simulink model "IFOC_SPVM"  (Simulink 8.3)
settings: Solver=ode23tb  SolverMode=SingleTasking  StartTime=0.0  StopTime=3
InitFcn:
  | assignin('base','Ts',[2e-6]); load power_acdrive_init;
undefined symbols (not defined in the file): Tlim
libraries: powerlib x7
Description:
  | The Model initialization function Callback automatically
  | 
  | sets the sample time  to 2e-6 sec.  and loads the initial
  | 
  | states vector xInitial. The initial state vector is saved in the
  | 
  | power_acdrive_init.mat file.
  | 
  | 
  | 
  | Check  the Initial state checkbox in the Simulation
  | 
  | parameters/Workspace I/O to start in steady state with a
  | 
  | speed of 120 rad/s and a torque of 0 N.m/s,
settings Model: Creator=Hoang Lehuy, Laval University  LastModifiedBy=Keshav  ExtModeTrigMode=oneshot  ExtModeArmWhenConnect=off  ExtModeAutoUpdateStatusClock=off
settings DataIOCC: LimitDataPoints=off  SaveFinalState=on  SaveFormat=StructureWithTime  SaveOutput=off  SaveTime=off  SignalLoggingName=sigsOut
settings OptimizationCC: BlockReduction=off  ExpressionDepthLimit=2147483647  InitFltsAndDblsToZero=on
settings DebuggingCC: SaveWithParameterizedLinksMsg=none  CheckExecutionContextPreStartOutputMsg=on  CheckExecutionContextRuntimeOutputMsg=on  SignalResolutionControl=TryResolveAllWithWarning  SolverPrmCheckMsg=none  MultiTaskDSMMsg=warning  MultiTaskCondExecSysMsg=none  FcnCallInpInsideContextMsg=UseLocalSettings  UnconnectedOutputMsg=none
settings HardwareCC: TargetUnknown=on
settings RTWCC: TemplateMakefile=grt_vc.tmf  IncludeERTFirstTime=on
settings GRTTargetCC: TargetFcnLib=ansi_tfl_tmw.mat

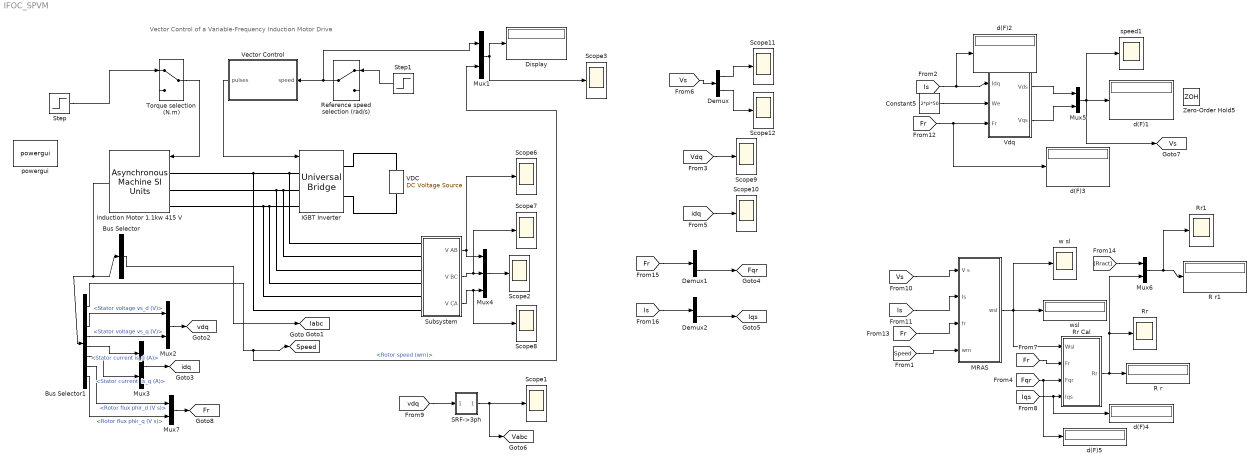
== system IFOC_SPVM ==
  note: Vector Control of a Variable-Frequency Induction Motor Drive
  Bus Selector : BusSelector  OutputSignals=Stator measurements.Stator current is_a (A),Stator measurements.Stator current is_b (A),Stator measurements.Stator current is_c (A)  OutputAsBus=on
  Bus Selector1 : BusSelector  OutputSignals="Mechanical.Rotor speed (wm),Mechanical.Electromagnetic torque Te (N*m),Stator measurements.Stator voltage vs_d (V),Stator measurements.Stator voltage vs_q (V),Stator measurements.Stator current is_d (A),Stator measurements.Stator current  is_q (A),Rotor measurements.Rotor flux phir_d (V s),Rotor measurements.Rotor flux phir_q (V s)"
  Constant5 : Constant  Value=2*pi*50
  Demux : Demux  Outputs=2
  Demux1 : Demux  Outputs=2
  Demux2 : Demux  Outputs=2
  Display : Display
  IGBT Inverter : powerlib/Power Electronics/Universal Bridge  Arms=3  SnubberResistance=1000  SnubberCapacitance=inf  Device=IGBT / Diodes  Ron=1e-3  Lon=0  ForwardVoltages="[  0.8  0.8  ]"  ForwardVoltage=.8  GTOparameters=[ 1e-6 , 1e-6 ]  IGBTparameters=[ 1e-6 , 2e-6 ]  Measurements=None  Measurements_2=None  converterType=Rectifier
  Induction Motor 1.1kw 415 V : powerlib/Machines/Asynchronous Machine SI Units  PresetModel=No  MechanicalLoad=Torque Tm  ShowDetailedParameters=on  RotorType=Squirrel-cage  ReferenceFrame=Synchronous  Units=SI  MeasurementBus=off  NominalParameters=[ 1.1e3,415, 50 ]  Stator=[6.03 0.0299]  Rotor=[12 0.0299]  Cage1=[ 0.022 0.226/377]  Cage2=[ 0.022 0.226/377]  Lm=0.4893  Mechanical="[0.011787  0.0027 2 ]"  PolePairs=2  InitialConditions="[ 1, 0 ,  0 , 0 , 0 , 0 , 0 , 0 ]"  SimulateSaturation=off  Saturation=[9.9249,19.6672,38.0377,51.3988,69.2824,105.1337,152.5532,214.2421,303.1917;230, 322, 414, 460, 506, 552, 598, 644, 690]  LoadFlowParameters=0  TsPowergui=0  TsBlock=-1  IterativeModel=Trapezoidal non iterative  Pmec=0
  MRAS : Subsystem  mask{Kp=100, Ki=50}
      mask prompts: Kp "Proportional Gain (Kp)"; Ki "Integral Gain (Ki)"
  Mux{1..3,5..7} (6 alike) : Mux  Inputs=2
  Mux4 : Mux  Inputs=3
  R r : Display
  R r1 : Display
  Reference speed selection (rad/s) : ManualSwitch
  Rr : Scope
      settings: TimeRange=2  YMin=0  YMax=1.4  SaveName=ScopeData2  MaxDataPoints=20000  Decimation=20
  Rr Cal : Subsystem
  Rr1 : Scope
      settings: TimeRange=2  YMin=12.14  YMax=12.17  SaveName=Resistance  MaxDataPoints=20000  Decimation=20
  SRF->3ph : Subsystem  AncestorBlock=plecslib_extras/Transformations/SRF->3ph  mask(Transformation SRF->3ph){}
      mask help:
      | Transforms a two-dimensional vector in the stationary reference frame into a three-phase signal:
      | [alpha beta] -> [a b c]
      mask Help: web(['file:///' fullfile(plecsdoc, 'alphabeta2abc.html')])
      mask Display: plot([0 100],[0 100], [0.5 3 4 4 5 4 3 1 0 0 1 4]*4+36,[7 7 6 3 2 3 2 2 3 4 5 5]*4, [0 1 3 4 4 3 1 0 0 0]*4+60,[6 7 7 6 3 2 2 3 2 10]*4, [4 3 1 0 0 1 3 4]*4+84,[6 7 7 6 3 2 2 3]*4, [5 3 1 0 0 1 3 5]*4,[7 2 2 3 6 7 7 2]*4+62, [0 0 1 3 4 4 3 2 3 4 4 3 1]*4+35,[0 8 9 9 8 7 6 6 6 5 3 2 2]*4+62 )
  Scope{1..3,6..12} (10 alike) : Scope
      Scope1 settings: TimeRange=0.5  YMin=-800  YMax=700  Decimation=20  SampleTime=5e-6
      Scope10 settings: TimeRange=0.5  YMin=1.5  YMax=4.5  SaveName=ScopeData9  Decimation=20  SampleTime=5e-6
      Scope11 settings: TimeRange=0.5  YMin=230  YMax=360  SaveName=ScopeData10  Decimation=20  SampleTime=5e-6
      Scope12 settings: TimeRange=0.5  YMin=-900  YMax=800  SaveName=ScopeData11  Decimation=20  SampleTime=5e-6
      Scope2 settings: TimeRange=0.5  YMin=-100  YMax=700  SaveName=ScopeData15  Decimation=20  SampleTime=5e-6
      Scope3 settings: TimeRange=0.5  YMin=-100  YMax=700  SaveName=ScopeData7  Decimation=20  SampleTime=5e-6
      Scope6 settings: TimeRange=0.5  YMin=-50  YMax=700  SaveName=ScopeData4  Decimation=20  SampleTime=5e-6
      Scope7 settings: TimeRange=0.5  YMin=-100  YMax=700  SaveName=ScopeData5  Decimation=20  SampleTime=5e-6
      Scope8 settings: TimeRange=0.5  YMin=-100  YMax=700  SaveName=ScopeData6  Decimation=20  SampleTime=5e-6
      Scope9 settings: TimeRange=0.5  YMin=-500  YMax=500  SaveName=ScopeData8  Decimation=20  SampleTime=5e-6
  Step : Step  Time=0  Before=7.5  After=7.5  SampleTime=0
  Step1 : Step  Time=0  Before=148.2  After=148.2  SampleTime=0
  Subsystem : Subsystem
  Torque selection (N.m) : ManualSwitch
  VDC : powerlib/Electrical Sources/DC Voltage Source  Description=source block  Amplitude=700  Measurements=None
      settings: AttributesFormatString=\n
  Vdq : Subsystem
  Vector Control : Subsystem
  Zero-Order Hold5 : ZeroOrderHold  SampleTime=0.1e-3
  d(F){1..5} (5 alike) : Display
  powergui : powerlib/powergui  Priority=1  SimulationMode=Continuous  SolverType=Tustin  SampleTime=50e-6  frequency=60  SPID=off  DisableSnubberDevices=off  DisableRonSwitches=off  DisableVfSwitches=off  SwTol=0  Interpol=off  DisplayEquations=off  Ts=0  methode=off  frequencyindice=50  Pbase=100e6  ErrMax=1e-4  Iterations=50  UnitsV=kV  UnitsW=MW  FunctionMessages=off  echomessages=off  HookPort=off  EnableUseOfTLC=off  x0status=blocks  RestoreLinks=warning  ResistiveCurrentMeasurement=off  Frange=[0:2:500]  Ylog=off  Xlog=on  ShowGrid=off  save=off  variable=ZData  structure=0  ZoomFFT=off  StartTime=0.0  cycles=1  DisplayStyle=1  fundamental=60  FreqAxis=off  MaxFrequency=1000  frequencyindicesteady=1  RmsSteady=1  display=off
  speed1 : Scope
      settings: TimeRange=2  YMin=-250  YMax=350  MaxDataPoints=20000  Decimation=20
  w sl : Scope
      settings: TimeRange=2  YMin=0  YMax=1.4  SaveName=ScopeData12  MaxDataPoints=20000  Decimation=20
  wsl : Display
  tag scope: Fqr=global, Fr=global, Iabc=global, Iqs=global, Speed=global, Vabc=global, Vs=global, idq=global, vdq=global
  wires:
  Torque selection (N.m)/1 -> Induction Motor 1.1kw 415 V/1
  Reference speed selection (rad/s)/1 -> Vector Control/1(speed), Mux1/1
  Induction Motor 1.1kw 415 V/1 -> Bus Selector1/1, Bus Selector/1
  Bus Selector/1 -> [Iabc]
  Bus Selector1/1 -> [Speed], Mux1/2  "<Rotor speed (wm)>"
  Mux1/1 -> Display/1, Scope3/1
  Vector Control/1(pulses) -> IGBT Inverter/1
  Mux2/1 -> [vdq]
  Mux3/1 -> [idq]
  Step1/1 -> Reference speed selection (rad/s)/1
  Step/1 -> Torque selection (N.m)/1
  Subsystem/1(V AB) -> Mux4/1, Scope6/1
  Subsystem/2(V BC) -> Mux4/2, Scope7/1
  Subsystem/3(V CA) -> Mux4/3, Scope8/1
  [Vdq] -> Scope9/1
  [idq] -> Scope10/1
  [Vs] -> Demux/1
  Demux/1 -> Scope11/1
  Demux/2 -> Scope12/1
  Mux4/1 -> Scope2/1
  Bus Selector1/3 -> Mux2/1  "<Stator voltage vs_d (V)>"
  Bus Selector1/4 -> Mux2/2  "<Stator voltage vs_q (V)>"
  Bus Selector1/5 -> Mux3/1  "<Stator current is_d (A)>"
  Bus Selector1/6 -> Mux3/2  "<Stator current  is_q (A)>"
  [Is] -> d(F)2/1, Vdq/1(Idq)
  Constant5/1 -> Vdq/2(We)
  Mux5/1 -> d(F)1/1, speed1/1, [Vs]
  Vdq/1(Vds) -> Mux5/1
  Vdq/2(Vqs) -> Mux5/2
  [Fr] -> d(F)3/1, Vdq/3(Fr)
  Bus Selector1/7 -> Mux7/1  "<Rotor flux phir_d (V s)>"
  Bus Selector1/8 -> Mux7/2  "<Rotor flux phir_q (V s)>"
  Mux7/1 -> [Fr]
  SRF->3ph/1(abc) -> Scope1/1, [Vabc]
  [vdq] -> SRF->3ph/1(alpha beta)
  [Vs] -> MRAS/1(V s)
  [Is] -> MRAS/2(Is)
  [Fr] -> MRAS/3(fr)
  MRAS/1(wsl) -> wsl/1, w sl/1, Rr Cal/1(Wsl)
  [Speed] -> MRAS/4(wm)
  [Fr] -> Rr Cal/2(Fr)
  [Fqr] -> Rr Cal/3(Fqr), d(F)5/1
  [Iqs] -> Rr Cal/4(Iqs), d(F)4/1
  Rr Cal/1(Rr) -> R r/1, Rr/1, Mux6/2
  [Rract] -> Mux6/1
  Mux6/1 -> R r1/1, Rr1/1
  [Fr] -> Demux1/1
  Demux1/2 -> [Fqr]
  [Is] -> Demux2/1
  Demux2/2 -> [Iqs]
  connections:
  IGBT Inverter/RConn2 -- VDC/LConn1
  Induction Motor 1.1kw 415 V/LConn3 -- IGBT Inverter/LConn3 -- Subsystem/LConn4 -- Subsystem/LConn5
  IGBT Inverter/LConn1 -- Subsystem/LConn1 -- Induction Motor 1.1kw 415 V/LConn1 -- Subsystem/LConn6
  IGBT Inverter/RConn1 -- VDC/RConn1
  Induction Motor 1.1kw 415 V/LConn2 -- IGBT Inverter/LConn2 -- Subsystem/LConn2 -- Subsystem/LConn3

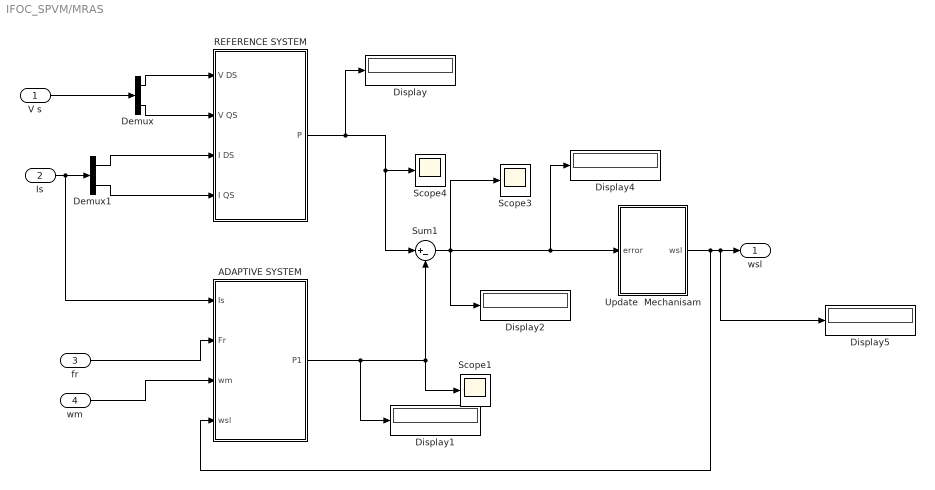
== system IFOC_SPVM/MRAS ==
  V s : Inport
  Is : Inport  Port=2
  fr : Inport  Port=3
  wm : Inport  Port=4
  ADAPTIVE SYSTEM : Subsystem
  Demux : Demux  Outputs=2
  Demux1 : Demux  Outputs=2
  Display{,1..2,4..5} (5 alike) : Display
  REFERENCE SYSTEM : Subsystem
  Scope1 : Scope
      settings: YMin=-1  YMax=1
  Scope3 : Scope
      settings: YMin=-1  YMax=1  SaveName=ScopeData16
  Scope4 : Scope
      settings: YMin=-1  YMax=1  SaveName=ScopeData4
  Sum1 : Sum  Inputs=|+-  SaturateOnIntegerOverflow=on  InputSameDT=on  OutDataTypeStr=Inherit: Same as first input
  Update  Mechanisam : Subsystem
  wsl : Outport
  wires:
  Demux/1 -> REFERENCE SYSTEM/1(V DS)
  Demux/2 -> REFERENCE SYSTEM/2(V QS)
  Demux1/1 -> REFERENCE SYSTEM/3(I DS)
  Demux1/2 -> REFERENCE SYSTEM/4(I QS)
  REFERENCE SYSTEM/1(P) -> Display/1, Sum1/1, Scope4/1
  ADAPTIVE SYSTEM/1(P1) -> Sum1/2, Scope1/1, Display1/1
  Is/1 -> Demux1/1, ADAPTIVE SYSTEM/1(Is)
  V s/1 -> Demux/1
  Sum1/1 -> Display2/1, Scope3/1, Update  Mechanisam/1(error), Display4/1
  fr/1 -> ADAPTIVE SYSTEM/2(Fr)
  wm/1 -> ADAPTIVE SYSTEM/3(wm)
  Update  Mechanisam/1(wsl) -> ADAPTIVE SYSTEM/4(wsl), wsl/1, Display5/1

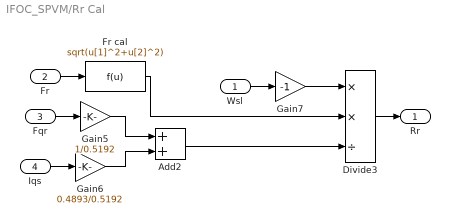
== system IFOC_SPVM/Rr Cal ==
  Wsl : Inport
  Fr : Inport  Port=2
  Fqr : Inport  Port=3
  Iqs : Inport  Port=4
  Add2 : Sum
  Divide3 : Product  Inputs=**/
  Fr cal : Fcn  Expr=sqrt(u[1]^2+u[2]^2)
  Gain5 : Gain  Gain=1/0.5192  SaturateOnIntegerOverflow=on  OutDataTypeStr=Inherit: Same as input  ParamDataTypeStr=Inherit: Same as input
  Gain6 : Gain  Gain=0.4893/0.5192  SaturateOnIntegerOverflow=on  OutDataTypeStr=Inherit: Same as input  ParamDataTypeStr=Inherit: Same as input
  Gain7 : Gain  Gain=-1  SaturateOnIntegerOverflow=on  OutDataTypeStr=Inherit: Same as input  ParamDataTypeStr=Inherit: Same as input
  Rr : Outport
  wires:
  Gain5/1 -> Add2/1
  Gain6/1 -> Add2/2
  Add2/1 -> Divide3/3
  Gain7/1 -> Divide3/1
  Fr cal/1 -> Divide3/2
  Fr/1 -> Fr cal/1
  Wsl/1 -> Gain7/1
  Divide3/1 -> Rr/1
  Fqr/1 -> Gain5/1
  Iqs/1 -> Gain6/1

== system IFOC_SPVM/SRF->3ph ==
  alpha beta : Inport  PortDimensions=2
  Mux : Mux  Inputs=3
  a : Fcn  Expr=u[1]
  b : Fcn  Expr=(-u[1]+sqrt(3)*u[2])/2
  c : Fcn  Expr=(-u[1]-sqrt(3)*u[2])/2
  abc : Outport
  wires:
  a/1 -> Mux/1
  b/1 -> Mux/2
  c/1 -> Mux/3
  Mux/1 -> abc/1
  alpha beta/1 -> b/1, a/1, c/1

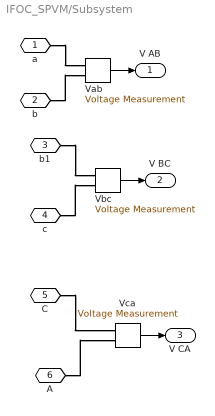
== system IFOC_SPVM/Subsystem ==
  Vab : powerlib/Measurements/Voltage Measurement  Tag=PoWeRsYsTeMmEaSuReMeNt  PhasorSimulation=off  OutputType=Magnitude  PSBequivalent=0
  Vbc : powerlib/Measurements/Voltage Measurement  Tag=PoWeRsYsTeMmEaSuReMeNt  PhasorSimulation=off  OutputType=Magnitude  PSBequivalent=0
  Vca : powerlib/Measurements/Voltage Measurement  Tag=PoWeRsYsTeMmEaSuReMeNt  PhasorSimulation=off  OutputType=Magnitude  PSBequivalent=0
  a : PMIOPort  Port=1  Side=Left
  b : PMIOPort  Port=2  Side=Left
  b1 : PMIOPort  Port=3  Side=Left
  c : PMIOPort  Port=4  Side=Left
  C : PMIOPort  Port=5  Side=Left
  A : PMIOPort  Port=6  Side=Left
  V AB : Outport
  V BC : Outport  Port=2
  V CA : Outport  Port=3
  wires:
  Vab/1 -> V AB/1
  Vbc/1 -> V BC/1
  Vca/1 -> V CA/1
  connections:
  a/RConn1 -- Vab/LConn1
  b/RConn1 -- Vab/LConn2
  b1/RConn1 -- Vbc/LConn1
  c/RConn1 -- Vbc/LConn2
  C/RConn1 -- Vca/LConn1
  A/RConn1 -- Vca/LConn2

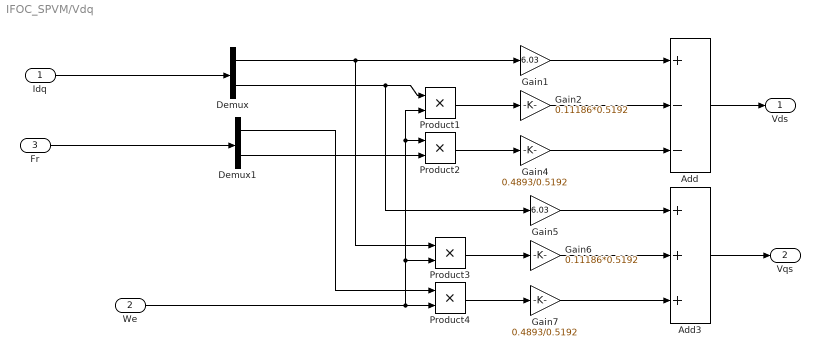
== system IFOC_SPVM/Vdq ==
  Idq : Inport
  We : Inport  Port=2
  Fr : Inport  Port=3
  Add : Sum  Inputs=+--
  Add3 : Sum  Inputs=+++
  Demux : Demux  Outputs=2
  Demux1 : Demux  Outputs=2
  Gain1 : Gain  Gain=6.03
  Gain2 : Gain  Gain=0.11186*0.5192
  Gain4 : Gain  Gain=0.4893/0.5192
  Gain5 : Gain  Gain=6.03
  Gain6 : Gain  Gain=0.11186*0.5192
  Gain7 : Gain  Gain=0.4893/0.5192
  Product{1..4} (4 alike) : Product  RndMeth=Zero
  Vds : Outport
  Vqs : Outport  Port=2
  wires:
  Idq/1 -> Demux/1
  Demux/1 -> Gain1/1, Product3/1
  Demux/2 -> Product1/1, Gain5/1
  Product1/1 -> Gain2/1
  Fr/1 -> Demux1/1
  Demux1/2 -> Product2/2
  Product2/1 -> Gain4/1
  Gain1/1 -> Add/1
  Gain2/1 -> Add/2
  Gain4/1 -> Add/3
  Product3/1 -> Gain6/1
  Product4/1 -> Gain7/1
  Demux1/1 -> Product4/1
  Gain5/1 -> Add3/1
  Gain6/1 -> Add3/2
  Gain7/1 -> Add3/3
  Add/1 -> Vds/1
  Add3/1 -> Vqs/1
  We/1 -> Product1/2, Product2/1, Product3/2, Product4/2

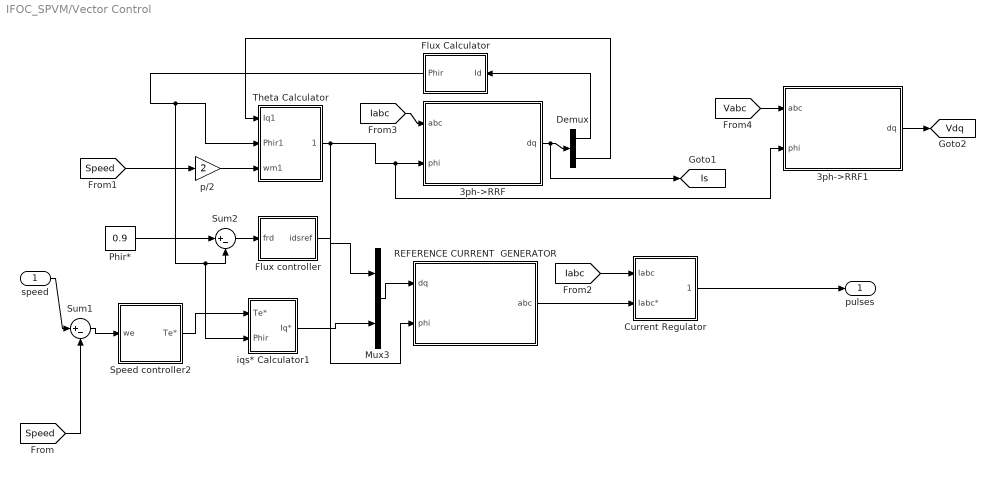
== system IFOC_SPVM/Vector Control ==
  speed : Inport
  " Flux controller" : Subsystem  Description=flux controller  mask(PI controller){Kp=10, Ki=100, MaskParam3=0}
      mask prompts: Kp "proportional gain"; Ki "Integral gain"; MaskParam3 "current limit"
      mask help: flux controller
      settings: ErrorFcn=flux controller
  3ph->RRF : Subsystem  mask(Transformation 3ph->RRF){}
      mask help:
      | Transforms a three-phase signal into a two-dimensional vector in a rotating reference frame. The rotation angle in radians of the rotating reference frame is determined by the second input:
      | [a b c], phi -> [d q]
      mask Help: web(['file:///' fullfile(plecsdoc, 'abc2dq.html')])
      mask Display:
      | plot(-30, -65, 150, 150)
      | plot([0 0 0 100],[0 100 50 50])
      | plot([0:5:100],[50+50.*sin([0:5:100]*2*pi/100)])
      | plot([0:5:100],[50+50.*sin(([0:5:100]*2*pi/100)+(2*pi/3))])
      | port_label('input',1,'ABC')
      | port_label('input',2,'Theta')
      | port_label('output',1,'DQ*')
  3ph->RRF1 : Subsystem  mask(Transformation 3ph->RRF){}
      mask help:
      | Transforms a three-phase signal into a two-dimensional vector in a rotating reference frame. The rotation angle in radians of the rotating reference frame is determined by the second input:
      | [a b c], phi -> [d q]
      mask Help: web(['file:///' fullfile(plecsdoc, 'abc2dq.html')])
      mask Display:
      | plot(-30, -65, 150, 150)
      | plot([0 0 0 100],[0 100 50 50])
      | plot([0:5:100],[50+50.*sin([0:5:100]*2*pi/100)])
      | plot([0:5:100],[50+50.*sin(([0:5:100]*2*pi/100)+(2*pi/3))])
      | port_label('input',1,'ABC')
      | port_label('input',2,'Theta')
      | port_label('output',1,'DQ*')
  Current Regulator : Subsystem  mask(Regulateur de courant a hysteresis){h=0.2}
      mask prompts: h "Hysteresis band (A)"
  Demux : Demux  Outputs=2
  Flux Calculator : Subsystem  mask(Flux Calcultation){}
      mask init:
      | NF=0.44572610323020e-6;
      | DF=[1 -0.99998715486734];
  Mux3 : Mux  Inputs=2
  Phir* : Constant  Value=0.9
  REFERENCE CURRENT  GENERATOR : Subsystem  mask(Transformation RRF->3ph){}
      mask help:
      | Transforms a two-dimensional vector in a rotating reference frame into a three-phase signal. The rotation angle in radians of the rotating reference frame is determined by the second input:
      | [d q], phi -> [a b c]
      mask Help: web(['file:///' fullfile(plecsdoc, 'dq2abc.html')])
      mask Display:
      | plot(-30, -65, 150, 150)
      | plot([0 0 0 100],[0 100 50 50])
      | plot([0:5:100],[50+50.*sin([0:5:100]*2*pi/100)])
      | plot([0:5:100],[50+50.*sin(([0:5:100]*2*pi/100)+(2*pi/3))])
      | plot([0:5:100],[50+50.*sin(([0:5:100]*2*pi/100)-(2*pi/3))])
      | port_label('input',1,'IDQ*')
      | port_label('input',2,'Theta')
      | port_label('output',1,'Iabc*')
  Speed controller2 : Subsystem  mask(PI controller){Kp=0.35, Ki=2.5, Tlim=0}
      mask prompts: Kp "Proportional gain (Kp)"; Ki "Integral gain (Ki)"; Tlim "Torque Limit"
      mask help: Proportional-Integral Speed Controller
      mask Display: plot(0,0,100,100,[35,35,65],[70,30,30],[35,65],[45,60])
  Sum1 : Sum  Inputs=|+-  SaturateOnIntegerOverflow=on  InputSameDT=on  OutDataTypeStr=Inherit: Same as first input
  Sum2 : Sum  Inputs=|+-  SaturateOnIntegerOverflow=on  InputSameDT=on  OutDataTypeStr=Inherit: Same as first input
  Theta Calculator : Subsystem
  iqs* Calculator1 : Subsystem
  p/2 : Gain  Gain=2  SaturateOnIntegerOverflow=on  OutDataTypeStr=Inherit: Same as input  ParamDataTypeStr=Inherit: Same as input
  pulses : Outport
  tag scope: Is=global, Vdq=global
  wires:
  Flux Calculator/1(Phir) -> Theta Calculator/2(Phir1), Sum2/2, iqs* Calculator1/2(Phir)
  [Iabc] -> Current Regulator/1(Iabc)
  [Iabc] -> 3ph->RRF/1(abc)
  Current Regulator/1(Pulses) -> pulses/1
  Sum1/1 -> Speed controller2/1(we)
  speed/1 -> Sum1/1
  [Speed] -> Sum1/2
  Speed controller2/1(Te*) -> iqs* Calculator1/1(Te*)
  Theta Calculator/1(theta1) -> 3ph->RRF/2(phi), 3ph->RRF1/2(phi), REFERENCE CURRENT  GENERATOR/2(phi)
  [Speed] -> p/2/1
  p/2/1 -> Theta Calculator/3(wm1)
  3ph->RRF/1(dq) -> Demux/1, [Is]
  Demux/1 -> Flux Calculator/1(Id)
  Demux/2 -> Theta Calculator/1(Iq1)
  " Flux controller"/1(idsref) -> Mux3/1
  iqs* Calculator1/1(Iq*) -> Mux3/2
  Mux3/1 -> REFERENCE CURRENT  GENERATOR/1(dq)
  REFERENCE CURRENT  GENERATOR/1(abc) -> Current Regulator/2(Iabc*)
  Phir*/1 -> Sum2/1
  Sum2/1 -> " Flux controller"/1(frd)
  [Vabc] -> 3ph->RRF1/1(abc)
  3ph->RRF1/1(dq) -> [Vdq]

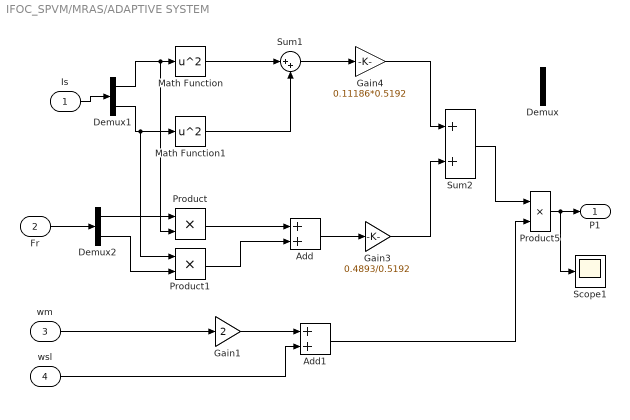
== system IFOC_SPVM/MRAS/ADAPTIVE SYSTEM ==
  Is : Inport
  Fr : Inport  Port=2
  wm : Inport  Port=3
  wsl : Inport  Port=4
  Add : Sum
  Add1 : Sum
  Demux : Demux  Outputs=2
  Demux1 : Demux  Outputs=2
  Demux2 : Demux  Outputs=2
  Gain1 : Gain  Gain=2  SaturateOnIntegerOverflow=on  OutDataTypeStr=Inherit: Same as input  ParamDataTypeStr=Inherit: Same as input
  Gain3 : Gain  Gain=0.4893/0.5192  SaturateOnIntegerOverflow=on  OutDataTypeStr=Inherit: Same as input  ParamDataTypeStr=Inherit: Same as input
  Gain4 : Gain  Gain=0.11186*0.5192  SaturateOnIntegerOverflow=on  OutDataTypeStr=Inherit: Same as input  ParamDataTypeStr=Inherit: Same as input
  Math Function : Math  Operator=square  SaturateOnIntegerOverflow=on
  Math Function1 : Math  Operator=square  SaturateOnIntegerOverflow=on
  Product : Product  RndMeth=Zero
  Product1 : Product  RndMeth=Zero
  Product5 : Product  SaturateOnIntegerOverflow=on  InputSameDT=on  OutDataTypeStr=Inherit: Same as first input
  Scope1 : Scope
      settings: YMin=-1  YMax=1  SaveName=ScopeData3
  Sum1 : Sum  Inputs=|++  SaturateOnIntegerOverflow=on  InputSameDT=on  OutDataTypeStr=Inherit: Same as first input
  Sum2 : Sum  SaturateOnIntegerOverflow=on  InputSameDT=on  OutDataTypeStr=Inherit: Same as first input
  P1 : Outport
  wires:
  Demux1/2 -> Math Function1/1, Product1/1
  Gain4/1 -> Sum2/1
  Sum1/1 -> Gain4/1
  Gain3/1 -> Sum2/2
  Sum2/1 -> Product5/1
  Product5/1 -> P1/1, Scope1/1
  Demux1/1 -> Math Function/1, Product/2
  Math Function/1 -> Sum1/1
  Math Function1/1 -> Sum1/2
  Is/1 -> Demux1/1
  Fr/1 -> Demux2/1
  Demux2/1 -> Product/1
  Demux2/2 -> Product1/2
  Product/1 -> Add/1
  Product1/1 -> Add/2
  Add/1 -> Gain3/1
  wm/1 -> Gain1/1
  Gain1/1 -> Add1/1
  wsl/1 -> Add1/2
  Add1/1 -> Product5/2

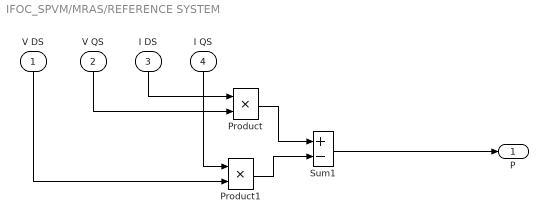
== system IFOC_SPVM/MRAS/REFERENCE SYSTEM ==
  V DS : Inport
  V QS : Inport  Port=2
  I DS : Inport  Port=3
  I QS : Inport  Port=4
  Product : Product  SaturateOnIntegerOverflow=on  OutDataTypeStr=Inherit: Same as first input
  Product1 : Product  SaturateOnIntegerOverflow=on  OutDataTypeStr=Inherit: Same as first input
  Sum1 : Sum  Inputs=+-  SaturateOnIntegerOverflow=on  InputSameDT=on  OutDataTypeStr=Inherit: Same as first input
  P : Outport
  wires:
  V QS/1 -> Product/2
  I DS/1 -> Product/1
  Product/1 -> Sum1/1
  V DS/1 -> Product1/2
  I QS/1 -> Product1/1
  Product1/1 -> Sum1/2
  Sum1/1 -> P/1

== system IFOC_SPVM/MRAS/Update  Mechanisam ==
  error : Inport
  PID Controller1 : Subsystem  AncestorBlock=simulink_extras/Additional Linear/PID Controller  mask(PID Controller){P=Kp, I=Ki}
      mask prompts: P "Proportional:"; I "Integral:"
      mask help:
      | Enter expressions for proportional, integral, and derivative terms.
      | P+I/s+Ds
      mask Help: This block implements a PID controller where parameters are entered for the Proportional, Integral and Derivative terms. Unmask this block to see how it works. The derivative term is implemented using a true derivative block.
      mask Display: disp('PI')
  Sum3 : Sum  Inputs=|+-  SaturateOnIntegerOverflow=on  InputSameDT=on  OutDataTypeStr=Inherit: Same as first input
  Unit Delay1 : UnitDelay  SampleTime=-1
  wsl : Outport
  wires:
  PID Controller1/1(Out_1) -> Sum3/1
  Sum3/1 -> Unit Delay1/1, wsl/1
  Unit Delay1/1 -> Sum3/2
  error/1 -> PID Controller1/1(In_1)

== system IFOC_SPVM/Vector Control/ Flux controller ==
  frd : Inport
  Gain : Gain  Gain=Ki  SaturateOnIntegerOverflow=on  OutDataTypeStr=Inherit: Same as input  ParamDataTypeStr=Inherit: Same as input
  Gain1 : Gain  Gain=Kp  SaturateOnIntegerOverflow=on  OutDataTypeStr=Inherit: Same as input  ParamDataTypeStr=Inherit: Same as input
  Integrator2 : Integrator  UpperSaturationLimit=Tlim  LowerSaturationLimit=-Tlim
  Sum2 : Sum  SaturateOnIntegerOverflow=on  InputSameDT=on  OutDataTypeStr=Inherit: Same as first input
  idsref : Outport  InitialOutput=0
  wires:
  Gain1/1 -> Sum2/1
  Gain/1 -> Integrator2/1
  frd/1 -> Gain/1, Gain1/1
  Sum2/1 -> idsref/1
  Integrator2/1 -> Sum2/2

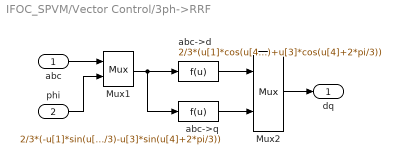
== system IFOC_SPVM/Vector Control/3ph->RRF ==
  abc : Inport  PortDimensions=3
  phi : Inport  Port=2  PortDimensions=1
  Mux1 : Mux  Inputs=2
  Mux2 : Mux  Inputs=2
  abc->d : Fcn  Expr=2/3*(u[1]*cos(u[4])+u[2]*cos(u[4]-2*pi/3)+u[3]*cos(u[4]+2*pi/3))
  abc->q : Fcn  Expr=2/3*(-u[1]*sin(u[4])-u[2]*sin(u[4]-2*pi/3)-u[3]*sin(u[4]+2*pi/3))
  dq : Outport
  wires:
  Mux1/1 -> abc->d/1, abc->q/1
  abc->q/1 -> Mux2/2
  abc->d/1 -> Mux2/1
  abc/1 -> Mux1/1
  phi/1 -> Mux1/2
  Mux2/1 -> dq/1

== system IFOC_SPVM/Vector Control/3ph->RRF1 ==
  abc : Inport  PortDimensions=3
  phi : Inport  Port=2  PortDimensions=1
  Mux1 : Mux  Inputs=2
  Mux2 : Mux  Inputs=2
  abc->d : Fcn  Expr=2/3*(u[1]*cos(u[4])+u[2]*cos(u[4]-2*pi/3)+u[3]*cos(u[4]+2*pi/3))
  abc->q : Fcn  Expr=2/3*(-u[1]*sin(u[4])-u[2]*sin(u[4]-2*pi/3)-u[3]*sin(u[4]+2*pi/3))
  dq : Outport
  wires:
  Mux2/1 -> dq/1
  phi/1 -> Mux1/2
  abc/1 -> Mux1/1
  abc->d/1 -> Mux2/1
  abc->q/1 -> Mux2/2
  Mux1/1 -> abc->q/1, abc->d/1

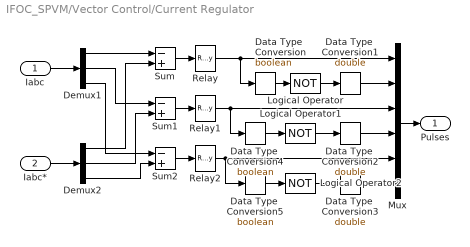
== system IFOC_SPVM/Vector Control/Current Regulator ==
  Iabc : Inport
  Iabc* : Inport  Port=2
  Data Type  Conversion : DataTypeConversion  OutDataTypeStr=boolean  SaturateOnIntegerOverflow=on  RndMeth=Zero
  Data Type  Conversion1 : DataTypeConversion  OutDataTypeStr=double  SaturateOnIntegerOverflow=on  RndMeth=Zero
  Data Type  Conversion2 : DataTypeConversion  OutDataTypeStr=double  SaturateOnIntegerOverflow=on  RndMeth=Zero
  Data Type  Conversion3 : DataTypeConversion  OutDataTypeStr=double  SaturateOnIntegerOverflow=on  RndMeth=Zero
  Data Type  Conversion4 : DataTypeConversion  OutDataTypeStr=boolean  SaturateOnIntegerOverflow=on  RndMeth=Zero
  Data Type  Conversion5 : DataTypeConversion  OutDataTypeStr=boolean  SaturateOnIntegerOverflow=on  RndMeth=Zero
  Demux1 : Demux  Outputs=3
  Demux2 : Demux  Outputs=3
  Logical Operator : Logic  Operator=NOT
  Logical Operator1 : Logic  Operator=NOT
  Logical Operator2 : Logic  Operator=NOT
  Mux : Mux  Inputs=6
  Relay : Relay  OnSwitchValue=h/2  OffSwitchValue=-h/2
  Relay1 : Relay  OnSwitchValue=h/2  OffSwitchValue=-h/2
  Relay2 : Relay  OnSwitchValue=h/2  OffSwitchValue=-h/2
  Sum : Sum  Inputs=-+  SaturateOnIntegerOverflow=on  InputSameDT=on  OutDataTypeStr=Inherit: Same as first input
  Sum1 : Sum  Inputs=-+  SaturateOnIntegerOverflow=on  InputSameDT=on  OutDataTypeStr=Inherit: Same as first input
  Sum2 : Sum  Inputs=-+  SaturateOnIntegerOverflow=on  InputSameDT=on  OutDataTypeStr=Inherit: Same as first input
  Pulses : Outport  InitialOutput=0
  wires:
  Sum/1 -> Relay/1
  Sum1/1 -> Relay1/1
  Demux1/1 -> Sum/1
  Demux1/2 -> Sum1/1
  Mux/1 -> Pulses/1
  Iabc/1 -> Demux1/1
  Sum2/1 -> Relay2/1
  Demux1/3 -> Sum2/1
  Demux2/3 -> Sum2/2
  Demux2/2 -> Sum1/2
  Demux2/1 -> Sum/2
  Iabc*/1 -> Demux2/1
  Relay/1 -> Mux/1, Data Type  Conversion/1
  Relay1/1 -> Mux/3, Data Type  Conversion4/1
  Relay2/1 -> Mux/5, Data Type  Conversion5/1
  Data Type  Conversion/1 -> Logical Operator/1
  Logical Operator/1 -> Data Type  Conversion1/1
  Data Type  Conversion1/1 -> Mux/2
  Logical Operator1/1 -> Data Type  Conversion2/1
  Data Type  Conversion2/1 -> Mux/4
  Logical Operator2/1 -> Data Type  Conversion3/1
  Data Type  Conversion3/1 -> Mux/6
  Data Type  Conversion4/1 -> Logical Operator1/1
  Data Type  Conversion5/1 -> Logical Operator2/1

== system IFOC_SPVM/Vector Control/Flux Calculator ==
  note: Phir = Lm *Id / (1 +Tr .s)
  note: Lm = 34.7 mH
  note: Lr = Ll'r +Lm = 0.013 +0.235= 0.248 H
  note: Tr = Lr / Rr = 0.1557 s
  Id : Inport
  Lm : Gain  Gain=0.4893  SaturateOnIntegerOverflow=on  OutDataTypeStr=Inherit: Same as input  ParamDataTypeStr=Inherit: Same as input
  Transfer Fcn : TransferFcn  Denominator=[0.08532 1]
  Phir : Outport
  wires:
  Transfer Fcn/1 -> Phir/1
  Id/1 -> Lm/1
  Lm/1 -> Transfer Fcn/1

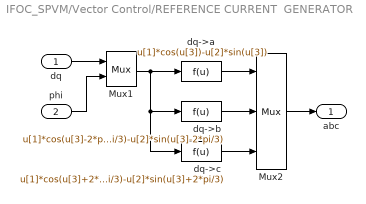
== system IFOC_SPVM/Vector Control/REFERENCE CURRENT  GENERATOR ==
  dq : Inport  PortDimensions=2
  phi : Inport  Port=2  PortDimensions=1
  Mux1 : Mux  Inputs=2
  Mux2 : Mux  Inputs=3
  dq->a : Fcn  Expr=u[1]*cos(u[3])-u[2]*sin(u[3])
  dq->b : Fcn  Expr=u[1]*cos(u[3]-2*pi/3)-u[2]*sin(u[3]-2*pi/3)
  dq->c : Fcn  Expr=u[1]*cos(u[3]+2*pi/3)-u[2]*sin(u[3]+2*pi/3)
  abc : Outport
  wires:
  dq->c/1 -> Mux2/3
  Mux2/1 -> abc/1
  dq->b/1 -> Mux2/2
  dq->a/1 -> Mux2/1
  Mux1/1 -> dq->c/1, dq->b/1, dq->a/1
  dq/1 -> Mux1/1
  phi/1 -> Mux1/2

== system IFOC_SPVM/Vector Control/Speed controller2 ==
  we : Inport
  Gain : Gain  Gain=Ki  SaturateOnIntegerOverflow=on  OutDataTypeStr=Inherit: Same as input  ParamDataTypeStr=Inherit: Same as input
  Gain1 : Gain  Gain=Kp  SaturateOnIntegerOverflow=on  OutDataTypeStr=Inherit: Same as input  ParamDataTypeStr=Inherit: Same as input
  Integrator2 : Integrator  UpperSaturationLimit=Tlim  LowerSaturationLimit=-Tlim
  Sum2 : Sum  SaturateOnIntegerOverflow=on  InputSameDT=on  OutDataTypeStr=Inherit: Same as first input
  Te* : Outport  InitialOutput=0
  wires:
  Integrator2/1 -> Sum2/2
  Sum2/1 -> Te*/1
  we/1 -> Gain1/1, Gain/1
  Gain/1 -> Integrator2/1
  Gain1/1 -> Sum2/1

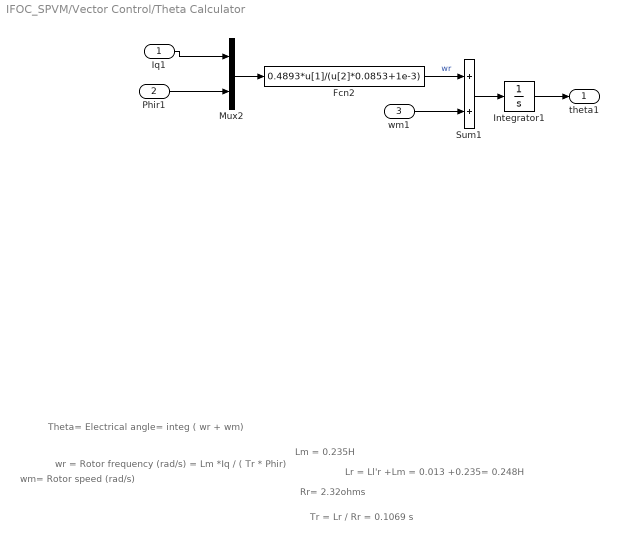
== system IFOC_SPVM/Vector Control/Theta Calculator ==
  note: Theta= Electrical angle= integ ( wr + wm)
  note: wr = Rotor frequency (rad/s) = Lm *Iq / ( Tr * Phir)
  note: Lm = 0.235H
  note: Rr= 2.32ohms
  note: Lr = Ll'r +Lm = 0.013 +0.235= 0.248H
  note: wm= Rotor speed (rad/s)
  note: Tr = Lr / Rr = 0.1069 s
  Iq1 : Inport
  Phir1 : Inport  Port=2
  wm1 : Inport  Port=3
  Fcn2 : Fcn  Expr=0.4893*u[1]/(u[2]*0.0853+1e-3)
  Integrator1 : Integrator
  Mux2 : Mux  Inputs=2
  Sum1 : Sum  SaturateOnIntegerOverflow=on  InputSameDT=on  OutDataTypeStr=Inherit: Same as first input
  theta1 : Outport  InitialOutput=0
  wires:
  Integrator1/1 -> theta1/1
  Sum1/1 -> Integrator1/1
  wm1/1 -> Sum1/2
  Fcn2/1 -> Sum1/1  "wr"
  Phir1/1 -> Mux2/2
  Iq1/1 -> Mux2/1
  Mux2/1 -> Fcn2/1

== system IFOC_SPVM/Vector Control/iqs* Calculator1 ==
  note: Iq= ( 2/3) * (2/p) * ( Lr/Lm) * (Te / Phir)
  note: Lm = 235 mH
  note: Lr = Ll'r +Lm = 0.013 +235=235.013 mH
  note: p= # of poles = 4
  note: Iq= 0.3537 * (Te / Phir)
  Te* : Inport
  Phir : Inport  Port=2
  Fcn : Fcn  Expr=u[1]*0.3537/(u[2]+1e-3)
  Mux1 : Mux  Inputs=2
  Iq* : Outport  InitialOutput=0
  wires:
  Phir/1 -> Mux1/2
  Te*/1 -> Mux1/1
  Mux1/1 -> Fcn/1
  Fcn/1 -> Iq*/1

== system IFOC_SPVM/MRAS/Update  Mechanisam/PID Controller1 ==
  In_1 : Inport
  Integral : TransferFcn  Numerator=[I]  Denominator=[1 0]
  Proportional : Gain  Gain=P  SaturateOnIntegerOverflow=on  OutDataTypeStr=Inherit: Same as input  ParamDataTypeStr=Inherit: Same as input
  Sum : Sum  SaturateOnIntegerOverflow=on  InputSameDT=on  OutDataTypeStr=Inherit: Same as first input
  Out_1 : Outport  InitialOutput=0
  wires:
  Sum/1 -> Out_1/1
  In_1/1 -> Proportional/1, Integral/1
  Integral/1 -> Sum/2
  Proportional/1 -> Sum/1
